simulink model "raven2_model"  (R2015b)
settings: Solver=ode5  SolverMode=SingleTasking  StartTime=0.0  StopTime=19.414  FixedStep=1e-3  RelTol=1e-3
values from neighbouring files (symbols this model uses):
  be1 = 1000*1    (= 1000)    [global_vars.m]
  be2 = 3*1380    (= 4140)    [global_vars.m]
  be3 = 1.0*400    (= 400)    [global_vars.m]
  F_cl1 = 0.505*1    (= 0.505)    [global_vars.m]
  F_cl2 = 0.49*1    (= 0.49)    [global_vars.m]
  F_cl3 = 0.53*10    (= 5.3)    [global_vars.m]
  F_vl1 = 0.00505*1.0    (= 0.00505)    [global_vars.m]
  F_vl2 = 0.0049*1    (= 0.0049)    [global_vars.m]
  F_vl3 = 0.0053*10    (= 0.053)    [global_vars.m]
  I1 = R1*[17.376 0.291 -0.374;0.291 11 -5.483;-0.374 -5.483 6.499]*1e-3*R1'+dI    [global_vars.m]
  I2 = R2*[81.579 0.773 0.762;0.773 44.329 37.973;0.762 37.973 37.686]*1e-3*R2'    [global_vars.m]
  I3 = R3*[2.908 -0.001 -0.066;-0.001 3.009 -0.009;-0.066 -0.009 0.355]*1e-3*R3'    [global_vars.m]
  Im1 = 2.847e-4*1.0    (= 0.0002847)    [global_vars.m]
  Im2 = 2.847e-4    (= 0.0002847)    [global_vars.m]
  Im3 = 2.847e-4    (= 0.0002847)    [global_vars.m]
  j1_r_max = 115/180*pi    (= 2.00712863979)    [joint_limits.m]
  j1_r_min = 10/180*pi    (= 0.174532925199)    [joint_limits.m]
  j2_r_max = 3*pi/4    (= 2.35619449019)    [joint_limits.m]
  j2_r_min = pi/4    (= 0.785398163397)    [joint_limits.m]
  j3_r_max = 520/1000    (= 0.52)    [joint_limits.m]
  j3_r_min = 260/1000    (= 0.26)    [joint_limits.m]
  jl_kd = 0.0    (= 0)    [global_vars.m]
  jl_kp = 0    [global_vars.m]
  kd_arm1 = 0.008*tr_1    (= 1.08957004405)    [global_vars.m]
  kd_arm2 = 20    [global_vars.m]
  kd_arm3 = 200    [global_vars.m]
  ke1 = 720e3    (= 720000)    [global_vars.m]
  ke2 = 3*88e3    (= 264000)    [global_vars.m]
  ke3 = 1*9.25e3    (= 9250)    [global_vars.m]
  ki_arm1 = 0    [global_vars.m]
  ki_arm2 = 0    [global_vars.m]
  ki_arm3 = 0    [global_vars.m]
  kp_arm1 = 0.3*tr_1    (= 40.858876652)    [global_vars.m]
  kp_arm2 = 500    [global_vars.m]
  kp_arm3 = 500    [global_vars.m]
  m1 = 0.503    [global_vars.m]
  m1_pos_ini = mpos1(1)    [initial_config.m]
  m1_vel_ini = mvel1(1)    [initial_config.m]
  m2 = 0.753    [global_vars.m]
  m2_pos_ini = mpos2(1)    [initial_config.m]
  m2_vel_ini = mvel2(1)    [initial_config.m]
  m3 = 0.407    [global_vars.m]
  m3_pos_ini = mpos3(1)    [initial_config.m]
  m3_vel_ini = mvel3(1)    [initial_config.m]
  N = 12.25    [global_vars.m]
  r_l1 = 63.095e-3    (= 0.063095)    [global_vars.m]
  r_l2 = 56.298e-3    (= 0.056298)    [global_vars.m]
  r_l3 = 1    [global_vars.m]
  r_mc1 = 5.675e-3    (= 0.005675)    [global_vars.m]
  r_mc2 = 5.675e-3    (= 0.005675)    [global_vars.m]
  r_mc3 = 5.675e-3    (= 0.005675)    [global_vars.m]
  tau_cm1 = 8.11e-2*0.9    (= 0.07299)    [global_vars.m]
  tau_cm2 = 4.11e-2*1.2    (= 0.04932)    [global_vars.m]
  tau_cm3 = 5.11e-2*2    (= 0.1022)    [global_vars.m]
  tau_vm1 = 1.9e-4*2    (= 0.00038)    [global_vars.m]
  tau_vm2 = 1.8e-4*12    (= 0.00216)    [global_vars.m]
  tau_vm3 = 7.1e-4*2    (= 0.00142)    [global_vars.m]
  theta1_0_r = pi/3    (= 1.0471975512)    [initial_config.m]    (also in main.m = random1*pi/180)
  theta1_d_r = 60*pi/180    (= 1.0471975512)    [main.m]
  theta2_0_r = pi/2    (= 1.57079632679)    [initial_config.m]    (also in main.m = random2*pi/180)
  theta2_d_r = 60*pi/180    (= 1.0471975512)    [main.m]
  theta3_0_r = 500/1000    (= 0.5)    [initial_config.m]    (also in main.m = random3/1000)
  theta3_d_r = 400/1000    (= 0.4)    [main.m]
libraries: mblibv1 x40, simulink x6
settings Model: Creator=raven_lab  LastModifiedBy=raven
settings DataIOCC: SaveFormat=Array
settings OptimizationCC: BlockReduction=off  BooleanDataType=off
settings DebuggingCC: SaveWithParameterizedLinksMsg=none  UnderspecifiedInitializationDetection=Classic  MergeDetectMultiDrivingBlocksExec=none  SignalResolutionControl=TryResolveAllWithWarning  MaskedZcDiagnostic=none  IgnoredZcDiagnostic=none
settings HardwareCC: ProdBitPerPointer=32  ProdLargestAtomicFloat=None  ProdIntDivRoundTo=Undefined  ProdEndianess=Unspecified  ProdWordSize=32  ProdHWDeviceType=32-bit Generic  TargetUnknown=on
settings GRTTargetCC: GeneratePreprocessorConditionals=Disable all
settings ConfigComp: CovModelRefEnable=Off
settings SimMechanicsCC: VisSampleTime=0.033  LastVizWinPosition=[1 41 1920 939]  CamPosition=[-0.0290778;0.260252;12.1482;]  CamTarget=[-0.0290778;0.260252;0.0240561;]  CamUpVector=[0;1;0;]  CamHeight=0.834655  VisBackgroundColor=[0.9;0.9;0.95;]  DefaultBodyColor=[1;0;0;]

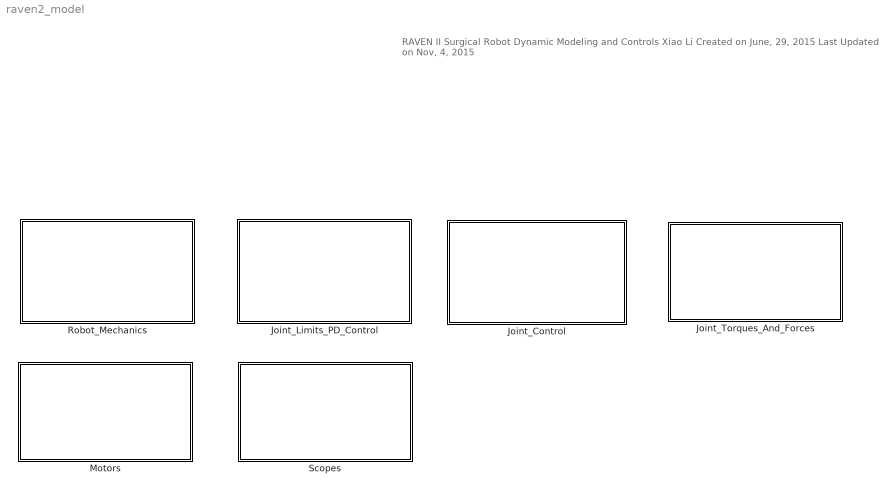
== system raven2_model ==
  note: RAVEN II Surgical Robot
      |
      | Dynamic Modeling and Controls
      |
      | Xiao Li
      |
      | Created on June, 29, 2015
      | Last Updated on Nov, 4, 2015
  Joint_Control : Subsystem
  Joint_Limits_PD_Control : Subsystem
  Joint_Torques_And_Forces : Subsystem
  Motors : Subsystem
  Robot_Mechanics : Subsystem
  Scopes : Subsystem

== system raven2_model/Joint_Control ==
  left_arm_control_command_signal : Subsystem
  right_arm_control_command_signal : Subsystem

== system raven2_model/Joint_Limits_PD_Control ==
  joint_r1_limit : Subsystem
  joint_r2_limit : Subsystem
  joint_r3_limit : Subsystem

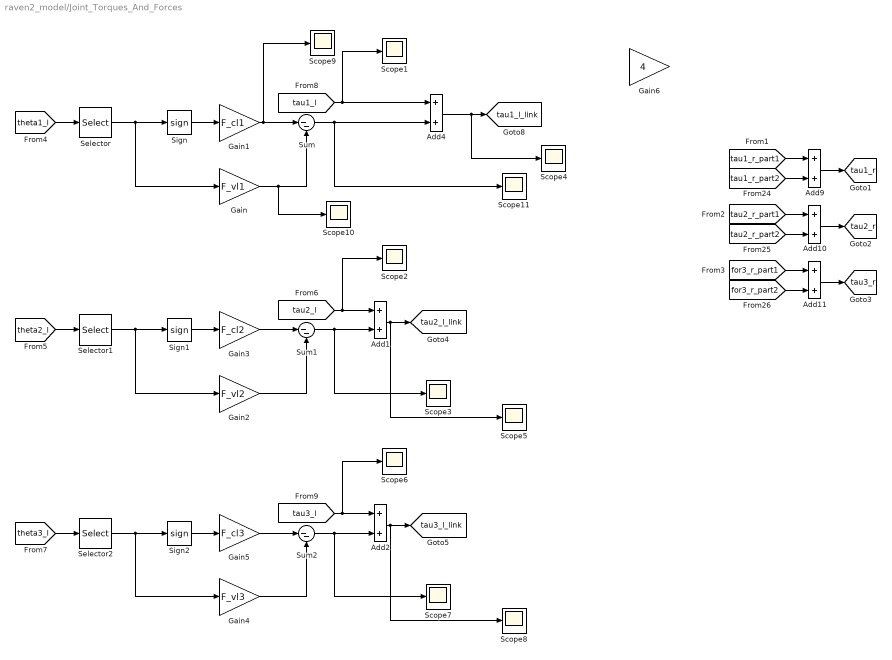
== system raven2_model/Joint_Torques_And_Forces ==
  Add{1..2,4,9..11} (6 alike) : Sum
  Gain : Gain  Gain=F_vl1
  Gain1 : Gain  Gain=F_cl1
  Gain2 : Gain  Gain=F_vl2
  Gain3 : Gain  Gain=F_cl2
  Gain4 : Gain  Gain=F_vl3
  Gain5 : Gain  Gain=F_cl3
  Gain6 : Gain  Gain=4
  Scope{1..11} (11 alike) : Scope
  Selector : Selector  InputPortWidth=2  IndexOptions=Index vector (dialog)  Indices=[2]  OutputSizes=1
  Selector1 : Selector  InputPortWidth=2  IndexOptions=Index vector (dialog)  Indices=[2]  OutputSizes=1
  Selector2 : Selector  InputPortWidth=2  IndexOptions=Index vector (dialog)  Indices=[2]  OutputSizes=1
  Sign : Signum
  Sign1 : Signum
  Sign2 : Signum
  Sum : Sum  Inputs=|--
  Sum1 : Sum  Inputs=|--
  Sum2 : Sum  Inputs=|--
  tag scope: tau1_l_link=global, tau1_r=global, tau2_l_link=global, tau2_r=global, tau3_l_link=global, tau3_r=global
  wires:
  Add4/1 -> Scope4/1, [tau1_l_link]
  [tau1_r_part2] -> Add9/2
  Add9/1 -> [tau1_r]
  [tau2_r_part2] -> Add10/2
  Add10/1 -> [tau2_r]
  [for3_r_part2] -> Add11/2
  Add11/1 -> [tau3_r]
  [tau1_r_part1] -> Add9/1
  [tau2_r_part1] -> Add10/1
  [for3_r_part1] -> Add11/1
  [theta1_l] -> Selector/1
  Sign/1 -> Gain1/1
  Selector/1 -> Gain/1, Sign/1
  Gain1/1 -> Scope9/1, Sum/1
  Gain/1 -> Scope10/1, Sum/2
  Sum/1 -> Scope11/1, Add4/2
  Add1/1 -> Scope5/1, [tau2_l_link]
  [theta2_l] -> Selector1/1
  Sign1/1 -> Gain3/1
  Selector1/1 -> Gain2/1, Sign1/1
  Gain3/1 -> Sum1/1
  Gain2/1 -> Sum1/2
  Sum1/1 -> Scope3/1, Add1/2
  [tau2_l] -> Scope2/1, Add1/1
  Add2/1 -> Scope8/1, [tau3_l_link]
  [theta3_l] -> Selector2/1
  Sign2/1 -> Gain5/1
  Selector2/1 -> Gain4/1, Sign2/1
  Gain5/1 -> Sum2/1
  Gain4/1 -> Sum2/2
  Sum2/1 -> Scope7/1, Add2/2
  [tau3_l] -> Scope6/1, Add2/1
  [tau1_l] -> Add4/1, Scope1/1

== system raven2_model/Motors ==
  Motor1 : Subsystem
  Motor2 : Subsystem
  Motor3 : Subsystem

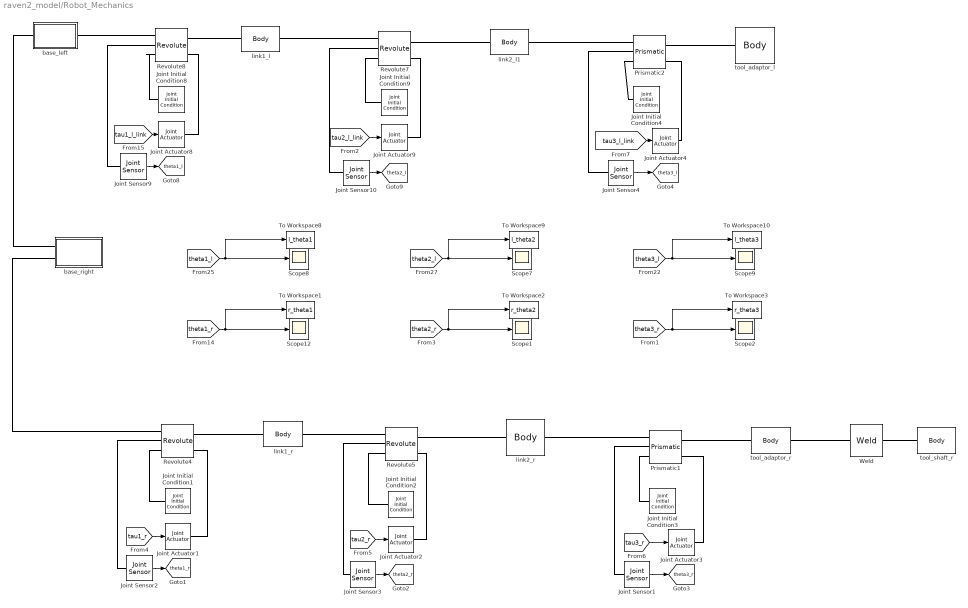
== system raven2_model/Robot_Mechanics ==
  Joint Actuator{1..2,8..9} (4 alike) : mblibv1/Sensors &  Actuators/Joint Actuator  UpdateFromCAD=off  PhysicalDomain=Mechanical  PortType=blob  ActuationStyle=Force  AngleUnits=deg  ArcVelocityUnits=deg/s  ArcAccelerationUnits=deg/s^2  CoordPositionUnits=m  VelocityUnits=m/s  AccelerationUnits=m/s^2  ForceUnits=N  TorqueUnits=N*m  ActiveIO=on  Width=1  DialogClass=MechanicalActuatorBlock  Primitive=R1  ReferenceFrame=Absolute (World)
  Joint Actuator3 : mblibv1/Sensors &  Actuators/Joint Actuator  UpdateFromCAD=off  PhysicalDomain=Mechanical  PortType=blob  ActuationStyle=Force  AngleUnits=deg  ArcVelocityUnits=deg/s  ArcAccelerationUnits=deg/s^2  CoordPositionUnits=m  VelocityUnits=m/s  AccelerationUnits=m/s^2  ForceUnits=N  TorqueUnits=N*m  ActiveIO=on  Width=1  DialogClass=MechanicalActuatorBlock  Primitive=P1  ReferenceFrame=Absolute (World)
  Joint Actuator4 : mblibv1/Sensors &  Actuators/Joint Actuator  UpdateFromCAD=off  PhysicalDomain=Mechanical  PortType=blob  ActuationStyle=Force  AngleUnits=deg  ArcVelocityUnits=deg/s  ArcAccelerationUnits=deg/s^2  CoordPositionUnits=m  VelocityUnits=m/s  AccelerationUnits=m/s^2  ForceUnits=N  TorqueUnits=N*m  ActiveIO=on  Width=1  DialogClass=MechanicalActuatorBlock  Primitive=P1  ReferenceFrame=Absolute (World)
  Joint Initial Condition1 : mblibv1/Sensors &  Actuators/Joint Initial Condition  UpdateFromCAD=off  LeftPortType=blob  RightPortType=blob  PhysicalDomain=mechanical  DialogClass=InitialConditionBlock  InitialConditions=P1$false$0$m$deg$0$m/s$deg/s#P2$false$0$m$deg$0$m/s$deg/s#P3$false$0$m$deg$0$m/s$deg/s#R1$true$theta1_0_r$m$rad$theta1_d_0_r$m/s$rad/s#R2$false$0$m$deg$0$m/s$deg/s#R3$false$0$m$deg$0$m/s$deg/s#S$false$0$m$deg$0$m/s$deg/s  P1PIC=0  P1VIC=0  P2PIC=0  P2VIC=0  P3PIC=0  P3VIC=0  R1PIC=theta1_0_r  R1VIC=theta1_d_0_r  R2PIC=0  R2VIC=0  R3PIC=0  R3VIC=0  SPIC=0  SVIC=0
  Joint Initial Condition2 : mblibv1/Sensors &  Actuators/Joint Initial Condition  UpdateFromCAD=off  LeftPortType=blob  RightPortType=blob  PhysicalDomain=mechanical  DialogClass=InitialConditionBlock  InitialConditions=P1$false$0$m$deg$0$m/s$deg/s#P2$false$0$m$deg$0$m/s$deg/s#P3$false$0$m$deg$0$m/s$deg/s#R1$true$theta2_0_r$m$rad$theta2_d_0_r$m/s$rad/s#R2$false$0$m$deg$0$m/s$deg/s#R3$false$0$m$deg$0$m/s$deg/s#S$false$0$m$deg$0$m/s$deg/s  P1PIC=0  P1VIC=0  P2PIC=0  P2VIC=0  P3PIC=0  P3VIC=0  R1PIC=theta2_0_r  R1VIC=theta2_d_0_r  R2PIC=0  R2VIC=0  R3PIC=0  R3VIC=0  SPIC=0  SVIC=0
  Joint Initial Condition3 : mblibv1/Sensors &  Actuators/Joint Initial Condition  UpdateFromCAD=off  LeftPortType=blob  RightPortType=blob  PhysicalDomain=mechanical  DialogClass=InitialConditionBlock  InitialConditions=P1$true$theta3_0_r$m$deg$theta3_d_0_r$m/s$deg/s#P2$false$0$m$deg$0$m/s$deg/s#P3$false$0$m$deg$0$m/s$deg/s#R1$false$theta2_0_r$m$rad$0$m/s$rad/s#R2$false$0$m$deg$0$m/s$deg/s#R3$false$0$m$deg$0$m/s$deg/s#S$false$0$m$deg$0$m/s$deg/s  P1PIC=theta3_0_r  P1VIC=theta3_d_0_r  P2PIC=0  P2VIC=0  P3PIC=0  P3VIC=0  R1PIC=0  R1VIC=0  R2PIC=0  R2VIC=0  R3PIC=0  R3VIC=0  SPIC=0  SVIC=0
  Joint Initial Condition4 : mblibv1/Sensors &  Actuators/Joint Initial Condition  UpdateFromCAD=off  LeftPortType=blob  RightPortType=blob  PhysicalDomain=mechanical  DialogClass=InitialConditionBlock  InitialConditions=P1$true$theta3_0_l$m$deg$theta3_d_0_l$m/s$deg/s#P2$false$0$m$deg$0$m/s$deg/s#P3$false$0$m$deg$0$m/s$deg/s#R1$false$theta2_0_r$m$rad$0$m/s$rad/s#R2$false$0$m$deg$0$m/s$deg/s#R3$false$0$m$deg$0$m/s$deg/s#S$false$0$m$deg$0$m/s$deg/s  P1PIC=theta3_0_l  P1VIC=theta3_d_0_l  P2PIC=0  P2VIC=0  P3PIC=0  P3VIC=0  R1PIC=0  R1VIC=0  R2PIC=0  R2VIC=0  R3PIC=0  R3VIC=0  SPIC=0  SVIC=0
  Joint Initial Condition8 : mblibv1/Sensors &  Actuators/Joint Initial Condition  UpdateFromCAD=off  LeftPortType=blob  RightPortType=blob  PhysicalDomain=mechanical  DialogClass=InitialConditionBlock  InitialConditions=P1$false$0$m$deg$0$m/s$deg/s#P2$false$0$m$deg$0$m/s$deg/s#P3$false$0$m$deg$0$m/s$deg/s#R1$true$theta1_0_l$m$rad$theta1_d_0_l$m/s$rad/s#R2$false$0$m$deg$0$m/s$deg/s#R3$false$0$m$deg$0$m/s$deg/s#S$false$0$m$deg$0$m/s$deg/s  P1PIC=0  P1VIC=0  P2PIC=0  P2VIC=0  P3PIC=0  P3VIC=0  R1PIC=theta1_0_l  R1VIC=theta1_d_0_l  R2PIC=0  R2VIC=0  R3PIC=0  R3VIC=0  SPIC=0  SVIC=0
  Joint Initial Condition9 : mblibv1/Sensors &  Actuators/Joint Initial Condition  UpdateFromCAD=off  LeftPortType=blob  RightPortType=blob  PhysicalDomain=mechanical  DialogClass=InitialConditionBlock  InitialConditions=P1$false$0$m$deg$0$m/s$deg/s#P2$false$0$m$deg$0$m/s$deg/s#P3$false$0$m$deg$0$m/s$deg/s#R1$true$theta2_0_l$m$rad$theta2_d_0_l$m/s$rad/s#R2$false$0$m$deg$0$m/s$deg/s#R3$false$0$m$deg$0$m/s$deg/s#S$false$0$m$deg$0$m/s$deg/s  P1PIC=0  P1VIC=0  P2PIC=0  P2VIC=0  P3PIC=0  P3VIC=0  R1PIC=theta2_0_l  R1VIC=theta2_d_0_l  R2PIC=0  R2VIC=0  R3PIC=0  R3VIC=0  SPIC=0  SVIC=0
  Joint Sensor1 : mblibv1/Sensors &  Actuators/Joint Sensor  UpdateFromCAD=off  PhysicalDomain=Mechanical  PortType=blob  Muxed=on  Pose=off  Angle=on  AngleUnits=deg  ArcVelocity=on  ArcVelocityUnits=deg/s  ArcAcceleration=off  ArcAccelerationUnits=deg/s^2  CoordPosition=on  CoordPositionUnits=m  Velocity=on  VelocityUnits=m/s  Acceleration=off  AccelerationUnits=m/s^2  Quaternion=on  QuaternionDT=off  QuaternionDDT=off  QuaternionUnits=off  OutputVector=[1]  ActiveIO=on  Width=2  DialogClass=MechanicalSensorBlock  Primitive=P1  Force=off  ForceUnits=N  Torque=off  TorqueUnits=N*m  ReferenceFrame=Absolute (World)  ReactionSensedSide=Base  ReactionReferenceFrame=Absolute (World)  ReactionForce=off  ReactionForceUnits=N  ReactionMoment=off  ReactionMomentUnits=N*m
  Joint Sensor{2..3,9..10} (4 alike) : mblibv1/Sensors &  Actuators/Joint Sensor  UpdateFromCAD=off  PhysicalDomain=Mechanical  PortType=blob  Muxed=on  Pose=off  Angle=on  AngleUnits=rad  ArcVelocity=on  ArcVelocityUnits=rad/s  ArcAcceleration=off  ArcAccelerationUnits=deg/s^2  CoordPosition=on  CoordPositionUnits=m  Velocity=off  VelocityUnits=m/s  Acceleration=off  AccelerationUnits=m/s^2  Quaternion=on  QuaternionDT=off  QuaternionDDT=off  QuaternionUnits=off  OutputVector=[1]  ActiveIO=on  Width=2  DialogClass=MechanicalSensorBlock  Primitive=R1  Force=off  ForceUnits=N  Torque=off  TorqueUnits=N*m  ReferenceFrame=Absolute (World)  ReactionSensedSide=Base  ReactionReferenceFrame=Absolute (World)  ReactionForce=off  ReactionForceUnits=N  ReactionMoment=off  ReactionMomentUnits=N*m
  Joint Sensor4 : mblibv1/Sensors &  Actuators/Joint Sensor  UpdateFromCAD=off  PhysicalDomain=Mechanical  PortType=blob  Muxed=on  Pose=off  Angle=on  AngleUnits=deg  ArcVelocity=on  ArcVelocityUnits=deg/s  ArcAcceleration=off  ArcAccelerationUnits=deg/s^2  CoordPosition=on  CoordPositionUnits=m  Velocity=on  VelocityUnits=m/s  Acceleration=off  AccelerationUnits=m/s^2  Quaternion=on  QuaternionDT=off  QuaternionDDT=off  QuaternionUnits=off  OutputVector=[1]  ActiveIO=on  Width=2  DialogClass=MechanicalSensorBlock  Primitive=P1  Force=off  ForceUnits=N  Torque=off  TorqueUnits=N*m  ReferenceFrame=Absolute (World)  ReactionSensedSide=Base  ReactionReferenceFrame=Absolute (World)  ReactionForce=off  ReactionForceUnits=N  ReactionMoment=off  ReactionMomentUnits=N*m
  Prismatic1 : mblibv1/Joints/Prismatic  LConnTagsString=__newl0|SA1|SA2  RConnTagsString=__newr0|SA1  UpdateFromCAD=on  NumSAPorts=3  CutJoint=off  MarkAsCut=off  Primitives=prismatic  PrimitiveProps=P1$World$-[0.601815,0,0.798636]$prismatic  DialogClass=JointBlock  P1Axis=-[0.601815,0,0.798636]
  Prismatic2 : mblibv1/Joints/Prismatic  LConnTagsString=__newl0|SA1|SA2  RConnTagsString=__newr0|SA1  UpdateFromCAD=on  NumSAPorts=3  CutJoint=off  MarkAsCut=off  Primitives=prismatic  PrimitiveProps=P1$World$-[0.920505,0,-0.390731]$prismatic  DialogClass=JointBlock  P1Axis=-[0.920505,0,-0.390731]
  Revolute4 : mblibv1/Joints/Revolute  LConnTagsString=__newl0|SA1|SA2  RConnTagsString=__newr0|SA1  UpdateFromCAD=on  NumSAPorts=3  CutJoint=off  MarkAsCut=off  Primitives=prismatic  PrimitiveProps=R1$World$[1,0,0]$revolute  DialogClass=JointBlock  R1Axis=[1,0,0]
  Revolute5 : mblibv1/Joints/Revolute  LConnTagsString=__newl0|SA1|SA2  RConnTagsString=__newr0|SA1  UpdateFromCAD=on  NumSAPorts=3  CutJoint=off  MarkAsCut=off  Primitives=prismatic  PrimitiveProps=R1$World$-[-0.258819,0,0.965926]$revolute  DialogClass=JointBlock  R1Axis=-[-0.258819,0,0.965926]
  Revolute7 : mblibv1/Joints/Revolute  LConnTagsString=__newl0|SA1|SA2  RConnTagsString=__newr0|SA1  UpdateFromCAD=on  NumSAPorts=3  CutJoint=off  MarkAsCut=off  Primitives=prismatic  PrimitiveProps=R1$World$-[-0.258819,0,0.965926]$revolute  DialogClass=JointBlock  R1Axis=-[-0.258819,0,0.965926]
  Revolute8 : mblibv1/Joints/Revolute  LConnTagsString=__newl0|SA1|SA2  RConnTagsString=__newr0|SA1  UpdateFromCAD=on  NumSAPorts=3  CutJoint=off  MarkAsCut=off  Primitives=prismatic  PrimitiveProps=R1$World$[1,0,0]$revolute  DialogClass=JointBlock  R1Axis=[1,0,0]
  Scope{1..2,7..9,12} (6 alike) : Scope
  To Workspace1 : ToWorkspace  VariableName=r_theta1  SaveFormat=Timeseries  SampleTime=-1
  To Workspace10 : ToWorkspace  VariableName=l_theta3  SaveFormat=Timeseries  SampleTime=-1
  To Workspace2 : ToWorkspace  VariableName=r_theta2  SaveFormat=Timeseries  SampleTime=-1
  To Workspace3 : ToWorkspace  VariableName=r_theta3  SaveFormat=Timeseries  SampleTime=-1
  To Workspace8 : ToWorkspace  VariableName=l_theta1  SaveFormat=Timeseries  SampleTime=-1
  To Workspace9 : ToWorkspace  VariableName=l_theta2  SaveFormat=Timeseries  SampleTime=-1
  Weld : mblibv1/Joints/Weld  LConnTagsString=__newl0  RConnTagsString=__newr0  UpdateFromCAD=off  NumSAPorts=0  CutJoint=off  MarkAsCut=off  Primitives=weld  PrimitiveProps=W$WORLD$[0 0 0]$weld  DialogClass=JointBlock  WAxis=[0 0 0]
  base_left : Subsystem
  base_right : Subsystem
  link1_l : mblibv1/Bodies/Body  LConnTagsString=CS3  RConnTagsString=CS2  UpdateFromCAD=on  DialogClass=MechanicalBodyBlock  Mass=m1  MassUnits=kg  InertiaUnits=kg*m^2  Inertia=I1  Shape=Cylinder  ShapeDims=[1 1]  ShapeUnits=m  ShapeUse=false  Density=1  DensityUnits=kg/m^3  DensityUse=false  GraphicsMode=GFXFILE  GraphicsFileName=full_robot - Sim_R2-Link1-L-1.STL  BodyColorSelMode=COLORPALETTE  BodyColor=[0.49412 0.49412 0.49412]  AttachedToCS=CS1  CG=Right$CG$[-0.215224 0.00717636 0.104721]$WORLD$WORLD$m$[1 0 0;0 -1 0;0 0 -1]$3x3 Transform$rad$WORLD$false$none  WorkingFrames=Right$CS1$[-0.278513 0 0]$WORLD$WORLD$m$[1 0 0;0 -1 0;0 0 -1]$3x3 Transform$rad$WORLD$false$none#Right$CS2$[-0.121275 0 0.143591]$WORLD$WORLD$m$[1 0 0;0 1 0;0 0 1]$3x3 Transform$rad$WORLD$true$none#Left$CS3$[-0.284078 0 0]$WORLD$WORLD$m$[1 0 0;0 1 0;0 0 1]$3x3 Transform$rad$WORLD$true$none  CGPos=[-0.215224 0.00717636 0.104721]  CGRot=[1 0 0;0 -1 0;0 0 -1]  CS0Pos=[]  CS0Rot=[]  CS1Pos=[-0.278513 0 0]  CS1Rot=[1 0 0;0 -1 0;0 0 -1]  CS2Pos=[-0.121275 0 0.143591]  CS2Rot=[1 0 0;0 1 0;0 0 1]  CS3Pos=[-0.284078 0 0]  CS3Rot=[1 0 0;0 1 0;0 0 1]  CS4Pos=[]  CS4Rot=[]  CS5Pos=[]  CS5Rot=[]  CS6Pos=[]  CS6Rot=[]  CS7Pos=[]  CS7Rot=[]  CS8Pos=[]  CS8Rot=[]  CS9Pos=[]  CS9Rot=[]  CS10Pos=[]  CS10Rot=[]  CS11Pos=[]  CS11Rot=[]  CS12Pos=[]  CS12Rot=[]  CS13Pos=[]  CS13Rot=[]  CS14Pos=[]  CS14Rot=[]  CS15Pos=[]  CS15Rot=[]  CS16Pos=[]  CS16Rot=[]  CS17Pos=[]  CS17Rot=[]  CS18Pos=[]  CS18Rot=[]  CS19Pos=[]  CS19Rot=[]  CS20Pos=[]  CS20Rot=[]
  link1_r : mblibv1/Bodies/Body  LConnTagsString=CS2  RConnTagsString=CS3  UpdateFromCAD=on  DialogClass=MechanicalBodyBlock  Mass=0.307878  MassUnits=kg  InertiaUnits=kg*m^2  Inertia=[0.000865925,5.99521e-06,-0.000512747;5.99521e-06,0.00142355,-6.10689e-06;-0.000512747,-6.10689e-06,0.000580565]  Shape=Cylinder  ShapeDims=[1 1]  ShapeUnits=m  ShapeUse=false  Density=1  DensityUnits=kg/m^3  DensityUse=false  GraphicsMode=GFXFILE  GraphicsFileName=full_robot - Sim_R2-Link1-R-1.STL  BodyColorSelMode=COLORPALETTE  BodyColor=[0.494118;0.494118;0.494118]  AttachedToCS=CS1  CG=Right$CG$[0.132424 -0.00717684 -0.104721]$WORLD$WORLD$m$[1 0 0;0 1 0;0 0 1]$3x3 Transform$rad$WORLD$false$none  WorkingFrames=Right$CS1$[0.195713 0 0]$WORLD$WORLD$m$[1 0 0;0 1 0;0 0 1]$3x3 Transform$rad$WORLD$false$none#Left$CS2$[0.200746 0 0]$WORLD$WORLD$m$[1 0 0;0 1 0;0 0 1]$3x3 Transform$rad$WORLD$true$none#Right$CS3$[0.0384751 0 -0.143591]$WORLD$WORLD$m$[1 0 0;0 1 0;0 0 1]$3x3 Transform$rad$WORLD$true$none  CGPos=[0.132424 -0.00717684 -0.104721]  CGRot=[1 0 0;0 1 0;0 0 1]  CS0Pos=[]  CS0Rot=[]  CS1Pos=[0.195713 0 0]  CS1Rot=[1 0 0;0 1 0;0 0 1]  CS2Pos=[0.200746 0 0]  CS2Rot=[1 0 0;0 1 0;0 0 1]  CS3Pos=[0.0384751 0 -0.143591]  CS3Rot=[1 0 0;0 1 0;0 0 1]  CS4Pos=[]  CS4Rot=[]  CS5Pos=[]  CS5Rot=[]  CS6Pos=[]  CS6Rot=[]  CS7Pos=[]  CS7Rot=[]  CS8Pos=[]  CS8Rot=[]  CS9Pos=[]  CS9Rot=[]  CS10Pos=[]  CS10Rot=[]  CS11Pos=[]  CS11Rot=[]  CS12Pos=[]  CS12Rot=[]  CS13Pos=[]  CS13Rot=[]  CS14Pos=[]  CS14Rot=[]  CS15Pos=[]  CS15Rot=[]  CS16Pos=[]  CS16Rot=[]  CS17Pos=[]  CS17Rot=[]  CS18Pos=[]  CS18Rot=[]  CS19Pos=[]  CS19Rot=[]  CS20Pos=[]  CS20Rot=[]
  link2_l1 : mblibv1/Bodies/Body  LConnTagsString=CS3  RConnTagsString=CS2  UpdateFromCAD=on  DialogClass=MechanicalBodyBlock  Mass=m2  MassUnits=kg  InertiaUnits=kg*m^2  Inertia=I2  Shape=Cylinder  ShapeDims=[1 1]  ShapeUnits=m  ShapeUse=false  Density=1  DensityUnits=kg/m^3  DensityUse=false  GraphicsMode=GFXFILE  GraphicsFileName=full_robot - Sim_R2-Link2-L-1.STL  BodyColorSelMode=COLORPALETTE  BodyColor=[0 0.44706 0.74118]  AttachedToCS=CS1  CG=Right$CG$[-0.30597 -0.00410333 0.168286]$WORLD$WORLD$m$[0.258819 -0.965926 0;0 0 1;-0.965926 -0.258819 0]$3x3 Transform$rad$WORLD$false$none  WorkingFrames=Right$CS1$[-0.162302 -0.0075 0.179517]$WORLD$WORLD$m$[0.258819 -0.965926 0;0 0 1;-0.965926 -0.258819 0]$3x3 Transform$rad$WORLD$false$none#Right$CS2$[-0.209463 0 0.0537709]$WORLD$WORLD$m$[1 0 0;0 1 0;0 0 1]$3x3 Transform$rad$WORLD$true$none#Left$CS3$[-0.121275 0 0.143591]$WORLD$WORLD$m$[1 0 0;0 1 0;0 0 1]$3x3 Transform$rad$WORLD$true$none  CGPos=[-0.30597 -0.00410333 0.168286]  CGRot=[0.258819 -0.965926 0;0 0 1;-0.965926 -0.258819 0]  CS0Pos=[]  CS0Rot=[]  CS1Pos=[-0.162302 -0.0075 0.179517]  CS1Rot=[0.258819 -0.965926 0;0 0 1;-0.965926 -0.258819 0]  CS2Pos=[-0.209463 0 0.0537709]  CS2Rot=[1 0 0;0 1 0;0 0 1]  CS3Pos=[-0.121275 0 0.143591]  CS3Rot=[1 0 0;0 1 0;0 0 1]  CS4Pos=[]  CS4Rot=[]  CS5Pos=[]  CS5Rot=[]  CS6Pos=[]  CS6Rot=[]  CS7Pos=[]  CS7Rot=[]  CS8Pos=[]  CS8Rot=[]  CS9Pos=[]  CS9Rot=[]  CS10Pos=[]  CS10Rot=[]  CS11Pos=[]  CS11Rot=[]  CS12Pos=[]  CS12Rot=[]  CS13Pos=[]  CS13Rot=[]  CS14Pos=[]  CS14Rot=[]  CS15Pos=[]  CS15Rot=[]  CS16Pos=[]  CS16Rot=[]  CS17Pos=[]  CS17Rot=[]  CS18Pos=[]  CS18Rot=[]  CS19Pos=[]  CS19Rot=[]  CS20Pos=[]  CS20Rot=[]
  link2_r : mblibv1/Bodies/Body  LConnTagsString=CS2  RConnTagsString=CS3  UpdateFromCAD=on  DialogClass=MechanicalBodyBlock  Mass=0.298287  MassUnits=kg  InertiaUnits=kg*m^2  Inertia=[0.00536881,-0.00335802,0.000118788;-0.00335802,0.00241011,0.000122449;0.000118788,0.000122449,0.00763968]  Shape=Cylinder  ShapeDims=[1 1]  ShapeUnits=m  ShapeUse=false  Density=1  DensityUnits=kg/m^3  DensityUse=false  GraphicsMode=GFXFILE  GraphicsFileName=full_robot - Sim_R2-Link2-R-1.STL  BodyColorSelMode=COLORPALETTE  BodyColor=[0;0.447059;0.741176]  AttachedToCS=CS1  CG=Right$CG$[-0.109127 -0.00410285 -0.257322]$WORLD$WORLD$m$[0.258819 -0.965926 0;0 0 1;-0.965926 -0.258819 0]$3x3 Transform$rad$WORLD$false$none  WorkingFrames=Right$CS1$[0.020908 -0.0075 -0.195217]$WORLD$WORLD$m$[0.258819 -0.965926 0;0 0 1;-0.965926 -0.258819 0]$3x3 Transform$rad$WORLD$false$none#Left$CS2$[0.0384751 0 -0.143591]$WORLD$WORLD$m$[1 0 0;0 1 0;0 0 1]$3x3 Transform$rad$WORLD$true$none#Right$CS3$[-0.0828081 0 -0.109899]$WORLD$WORLD$m$[1 0 0;0 1 0;0 0 1]$3x3 Transform$rad$WORLD$true$none  CGPos=[-0.109127 -0.00410285 -0.257322]  CGRot=[0.258819 -0.965926 0;0 0 1;-0.965926 -0.258819 0]  CS0Pos=[]  CS0Rot=[]  CS1Pos=[0.020908 -0.0075 -0.195217]  CS1Rot=[0.258819 -0.965926 0;0 0 1;-0.965926 -0.258819 0]  CS2Pos=[0.0384751 0 -0.143591]  CS2Rot=[1 0 0;0 1 0;0 0 1]  CS3Pos=[-0.0828081 0 -0.109899]  CS3Rot=[1 0 0;0 1 0;0 0 1]  CS4Pos=[]  CS4Rot=[]  CS5Pos=[]  CS5Rot=[]  CS6Pos=[]  CS6Rot=[]  CS7Pos=[]  CS7Rot=[]  CS8Pos=[]  CS8Rot=[]  CS9Pos=[]  CS9Rot=[]  CS10Pos=[]  CS10Rot=[]  CS11Pos=[]  CS11Rot=[]  CS12Pos=[]  CS12Rot=[]  CS13Pos=[]  CS13Rot=[]  CS14Pos=[]  CS14Rot=[]  CS15Pos=[]  CS15Rot=[]  CS16Pos=[]  CS16Rot=[]  CS17Pos=[]  CS17Rot=[]  CS18Pos=[]  CS18Rot=[]  CS19Pos=[]  CS19Rot=[]  CS20Pos=[]  CS20Rot=[]
  tool_adaptor_l : mblibv1/Bodies/Body  RConnTagsString=CS3  UpdateFromCAD=on  DialogClass=MechanicalBodyBlock  Mass=m3  MassUnits=kg  InertiaUnits=kg*m^2  Inertia=I3  Shape=Cylinder  ShapeDims=[1 1]  ShapeUnits=m  ShapeUse=false  Density=1  DensityUnits=kg/m^3  DensityUse=false  GraphicsMode=GFXFILE  GraphicsFileName=full_robot - tool_adaptor_r-3.STL  BodyColorSelMode=COLORPALETTE  BodyColor=[1 1 0]  AttachedToCS=CS1  CG=Right$CG$[-0.0750172 0.000150527 0.0170169]$WORLD$WORLD$m$[0 -0.920505 -0.390731;-1 0 0;0 0.390731 -0.920505]$3x3 Transform$rad$WORLD$false$none  WorkingFrames=Right$CS1$[0.0371929 0.0207212 0.0861524]$WORLD$WORLD$m$[0 -0.920505 -0.390731;-1 0 0;0 0.390731 -0.920505]$3x3 Transform$rad$WORLD$false$none#Left$CS2$[-0.0247371 0 -0.0246407]$WORLD$WORLD$m$[1 0 0;0 1 0;0 0 1]$3x3 Transform$rad$WORLD$false$none#Right$CS3$[-0.0303586 0 -0.0222545]$WORLD$WORLD$m$[1 0 0;0 1 0;0 0 1]$3x3 Transform$rad$WORLD$true$none  CGPos=[-0.0750172 0.000150527 0.0170169]  CGRot=[0 -0.920505 -0.390731;-1 0 0;0 0.390731 -0.920505]  CS0Pos=[]  CS0Rot=[]  CS1Pos=[0.0371929 0.0207212 0.0861524]  CS1Rot=[0 -0.920505 -0.390731;-1 0 0;0 0.390731 -0.920505]  CS2Pos=[-0.0247371 0 -0.0246407]  CS2Rot=[1 0 0;0 1 0;0 0 1]  CS3Pos=[-0.0303586 0 -0.0222545]  CS3Rot=[1 0 0;0 1 0;0 0 1]  CS4Pos=[]  CS4Rot=[]  CS5Pos=[]  CS5Rot=[]  CS6Pos=[]  CS6Rot=[]  CS7Pos=[]  CS7Rot=[]  CS8Pos=[]  CS8Rot=[]  CS9Pos=[]  CS9Rot=[]  CS10Pos=[]  CS10Rot=[]  CS11Pos=[]  CS11Rot=[]  CS12Pos=[]  CS12Rot=[]  CS13Pos=[]  CS13Rot=[]  CS14Pos=[]  CS14Rot=[]  CS15Pos=[]  CS15Rot=[]  CS16Pos=[]  CS16Rot=[]  CS17Pos=[]  CS17Rot=[]  CS18Pos=[]  CS18Rot=[]  CS19Pos=[]  CS19Rot=[]  CS20Pos=[]  CS20Rot=[]
  tool_adaptor_r : mblibv1/Bodies/Body  LConnTagsString=CS3  RConnTagsString=CS2  UpdateFromCAD=on  DialogClass=MechanicalBodyBlock  Mass=0.17959  MassUnits=kg  InertiaUnits=kg*m^2  Inertia=1e3*[1.75049e-07,2.47824e-09,4.64456e-10;2.47824e-09,7.90471e-08,4.11989e-09;4.64456e-10,4.11989e-09,1.78166e-07]  Shape=Cylinder  ShapeDims=[1 1]  ShapeUnits=m  ShapeUse=false  Density=1  DensityUnits=kg/m^3  DensityUse=false  GraphicsMode=GFXFILE  GraphicsFileName=full_robot - tool_adaptor_r-2.STL  BodyColorSelMode=COLORPALETTE  BodyColor=[0;1;0]  AttachedToCS=CS1  CG=Right$CG$[0.0152555 -0.000150527 -0.0108364]$WORLD$WORLD$m$[0 -0.601815 -0.798636;1 0 0;0 -0.798636 0.601815]$3x3 Transform$rad$WORLD$false$none  WorkingFrames=Right$CS1$[0.147 -0.0207212 -0.0146044]$WORLD$WORLD$m$[0 -0.601815 -0.798636;1 0 0;0 -0.798636 0.601815]$3x3 Transform$rad$WORLD$false$none#Right$CS2$[0.0379706 0 0.0503802]$WORLD$WORLD$m$[1 0 0;0 1 0;0 0 1]$3x3 Transform$rad$WORLD$true$none#Left$CS3$[0.0342953 0 0.0455029]$WORLD$WORLD$m$[1 0 0;0 1 0;0 0 1]$3x3 Transform$rad$WORLD$true$none  CGPos=[0.0152555 -0.000150527 -0.0108364]  CGRot=[0 -0.601815 -0.798636;1 0 0;0 -0.798636 0.601815]  CS0Pos=[]  CS0Rot=[]  CS1Pos=[0.147 -0.0207212 -0.0146044]  CS1Rot=[0 -0.601815 -0.798636;1 0 0;0 -0.798636 0.601815]  CS2Pos=[0.0379706 0 0.0503802]  CS2Rot=[1 0 0;0 1 0;0 0 1]  CS3Pos=[0.0342953 0 0.0455029]  CS3Rot=[1 0 0;0 1 0;0 0 1]  CS4Pos=[]  CS4Rot=[]  CS5Pos=[]  CS5Rot=[]  CS6Pos=[]  CS6Rot=[]  CS7Pos=[]  CS7Rot=[]  CS8Pos=[]  CS8Rot=[]  CS9Pos=[]  CS9Rot=[]  CS10Pos=[]  CS10Rot=[]  CS11Pos=[]  CS11Rot=[]  CS12Pos=[]  CS12Rot=[]  CS13Pos=[]  CS13Rot=[]  CS14Pos=[]  CS14Rot=[]  CS15Pos=[]  CS15Rot=[]  CS16Pos=[]  CS16Rot=[]  CS17Pos=[]  CS17Rot=[]  CS18Pos=[]  CS18Rot=[]  CS19Pos=[]  CS19Rot=[]  CS20Pos=[]  CS20Rot=[]
  tool_shaft_r : mblibv1/Bodies/Body  LConnTagsString=CS3  UpdateFromCAD=on  DialogClass=MechanicalBodyBlock  Mass=0.031894  MassUnits=kg  InertiaUnits=kg*m^2  Inertia=[0.000438543,1.00962e-12,-5.16101e-11;1.00962e-12,0.000438544,-2.93392e-12;-5.16101e-11,-2.93392e-12,3.98541e-07]  Shape=Cylinder  ShapeDims=[1 1]  ShapeUnits=m  ShapeUse=false  Density=1  DensityUnits=kg/m^3  DensityUse=false  GraphicsMode=GFXFILE  GraphicsFileName=full_robot - Sim_ToolShaft-1.STL  BodyColorSelMode=COLORPALETTE  BodyColor=[0.79216 0.81961 0.93333]  AttachedToCS=CS1  CG=Right$CG$[0.160168 -1.00252e-08 0.212541]$WORLD$WORLD$m$[0 0.798636 -0.601815;1 0 0;0 -0.601815 -0.798636]$3x3 Transform$rad$WORLD$false$none  WorkingFrames=Right$CS1$[0.278697 0 0.369834]$WORLD$WORLD$m$[0 0.798636 -0.601815;1 0 0;0 -0.601815 -0.798636]$3x3 Transform$rad$WORLD$false$none#Right$CS2$[0.28303 0.0011 0.375585]$WORLD$WORLD$m$[1 0 0;0 1 0;0 0 1]$3x3 Transform$rad$WORLD$false$none#Left$CS3$[0.0379706 0 0.0503802]$WORLD$WORLD$m$[1 0 0;0 1 0;0 0 1]$3x3 Transform$rad$WORLD$true$none  CGPos=[0.160168 -1.00252e-08 0.212541]  CGRot=[0 0.798636 -0.601815;1 0 0;0 -0.601815 -0.798636]  CS0Pos=[]  CS0Rot=[]  CS1Pos=[0.278697 0 0.369834]  CS1Rot=[0 0.798636 -0.601815;1 0 0;0 -0.601815 -0.798636]  CS2Pos=[0.28303 0.0011 0.375585]  CS2Rot=[1 0 0;0 1 0;0 0 1]  CS3Pos=[0.0379706 0 0.0503802]  CS3Rot=[1 0 0;0 1 0;0 0 1]  CS4Pos=[]  CS4Rot=[]  CS5Pos=[]  CS5Rot=[]  CS6Pos=[]  CS6Rot=[]  CS7Pos=[]  CS7Rot=[]  CS8Pos=[]  CS8Rot=[]  CS9Pos=[]  CS9Rot=[]  CS10Pos=[]  CS10Rot=[]  CS11Pos=[]  CS11Rot=[]  CS12Pos=[]  CS12Rot=[]  CS13Pos=[]  CS13Rot=[]  CS14Pos=[]  CS14Rot=[]  CS15Pos=[]  CS15Rot=[]  CS16Pos=[]  CS16Rot=[]  CS17Pos=[]  CS17Rot=[]  CS18Pos=[]  CS18Rot=[]  CS19Pos=[]  CS19Rot=[]  CS20Pos=[]  CS20Rot=[]
  tag scope: theta1_l=global, theta1_r=global, theta2_l=global, theta2_r=global, theta3_l=global, theta3_r=global
  wires:
  [tau1_r] -> Joint Actuator1/1
  Joint Sensor3/1 -> [theta2_r]
  Joint Sensor1/1 -> [theta3_r]
  [theta1_r] -> To Workspace1/1, Scope12/1
  [theta2_r] -> To Workspace2/1, Scope1/1
  [tau2_r] -> Joint Actuator2/1
  Joint Sensor2/1 -> [theta1_r]
  [theta3_r] -> To Workspace3/1, Scope2/1
  [tau3_r] -> Joint Actuator3/1
  [theta1_l] -> To Workspace8/1, Scope8/1
  [theta2_l] -> To Workspace9/1, Scope7/1
  [theta3_l] -> To Workspace10/1, Scope9/1
  Joint Sensor9/1 -> [theta1_l]
  [tau1_l_link] -> Joint Actuator8/1
  Joint Sensor10/1 -> [theta2_l]
  [tau2_l_link] -> Joint Actuator9/1
  [tau3_l_link] -> Joint Actuator4/1
  Joint Sensor4/1 -> [theta3_l]
  connections:
  link1_l/RConn1 -- Revolute7/LConn1
  base_right/LConn2 -- Revolute4/LConn1
  base_left/RConn1 -- Revolute8/LConn1
  Revolute5/LConn1 -- link1_r/RConn1
  Revolute8/RConn1 -- link1_l/LConn1
  Weld/LConn1 -- tool_adaptor_r/RConn1
  Weld/RConn1 -- tool_shaft_r/LConn1
  link2_r/LConn1 -- Revolute5/RConn1
  Prismatic1/RConn1 -- tool_adaptor_r/LConn1
  link2_r/RConn1 -- Prismatic1/LConn1
  base_right/LConn1 -- base_left/LConn1
  Revolute4/LConn2 -- Joint Sensor2/LConn1
  Prismatic1/LConn2 -- Joint Sensor1/LConn1
  Revolute4/RConn1 -- link1_r/LConn1
  Revolute5/RConn2 -- Joint Actuator2/RConn1
  Prismatic1/RConn2 -- Joint Actuator3/RConn1
  Revolute5/LConn3 -- Joint Initial Condition2/RConn1
  Revolute4/LConn3 -- Joint Initial Condition1/RConn1
  Revolute5/LConn2 -- Joint Sensor3/LConn1
  Revolute4/RConn2 -- Joint Actuator1/RConn1
  Prismatic1/LConn3 -- Joint Initial Condition3/RConn1
  Revolute8/LConn3 -- Joint Initial Condition8/RConn1
  Revolute8/RConn2 -- Joint Actuator8/RConn1
  Revolute7/RConn2 -- Joint Actuator9/RConn1
  Revolute7/LConn2 -- Joint Sensor10/LConn1
  Revolute7/LConn3 -- Joint Initial Condition9/RConn1
  Revolute8/LConn2 -- Joint Sensor9/LConn1
  Prismatic2/RConn2 -- Joint Actuator4/RConn1
  Prismatic2/RConn1 -- tool_adaptor_l/RConn1
  Prismatic2/LConn2 -- Joint Sensor4/LConn1
  Prismatic2/LConn3 -- Joint Initial Condition4/RConn1
  Revolute7/RConn1 -- link2_l1/LConn1
  link2_l1/RConn1 -- Prismatic2/LConn1

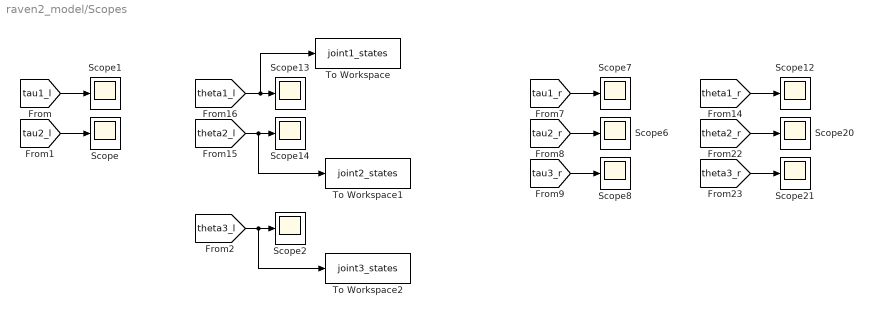
== system raven2_model/Scopes ==
  Scope{,1..2,6..8,12..14,20..21} (11 alike) : Scope
  To Workspace : ToWorkspace  VariableName=joint1_states  SaveFormat=Timeseries  SampleTime=-1
  To Workspace1 : ToWorkspace  VariableName=joint2_states  SaveFormat=Timeseries  SampleTime=-1
  To Workspace2 : ToWorkspace  VariableName=joint3_states  SaveFormat=Timeseries  SampleTime=-1
  wires:
  [tau2_l] -> Scope/1
  [tau1_l] -> Scope1/1
  [tau2_r] -> Scope6/1
  [tau1_r] -> Scope7/1
  [tau3_r] -> Scope8/1
  [theta1_r] -> Scope12/1
  [theta1_l] -> To Workspace/1, Scope13/1
  [theta2_l] -> To Workspace1/1, Scope14/1
  [theta2_r] -> Scope20/1
  [theta3_r] -> Scope21/1
  [theta3_l] -> To Workspace2/1, Scope2/1

== system raven2_model/Joint_Control/left_arm_control_command_signal ==

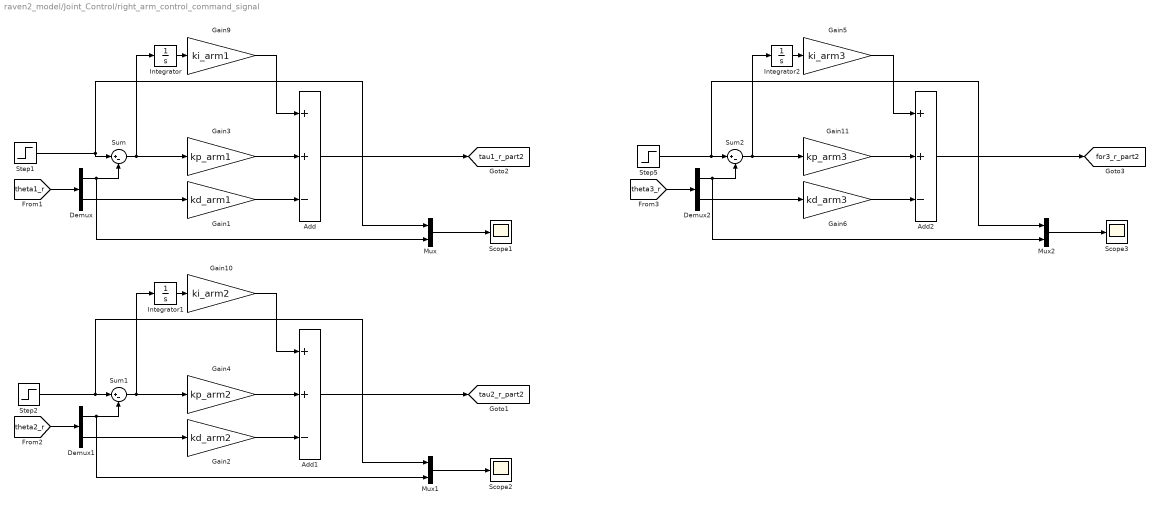
== system raven2_model/Joint_Control/right_arm_control_command_signal ==
  Add : Sum  Inputs=++-
  Add1 : Sum  Inputs=++-
  Add2 : Sum  Inputs=++-
  Demux : Demux  Outputs=2
  Demux1 : Demux  Outputs=2
  Demux2 : Demux  Outputs=2
  Gain1 : Gain  Gain=kd_arm1
  Gain10 : Gain  Gain=ki_arm2
  Gain11 : Gain  Gain=kp_arm3
  Gain2 : Gain  Gain=kd_arm2
  Gain3 : Gain  Gain=kp_arm1
  Gain4 : Gain  Gain=kp_arm2
  Gain5 : Gain  Gain=ki_arm3
  Gain6 : Gain  Gain=kd_arm3
  Gain9 : Gain  Gain=ki_arm1
  Integrator : Integrator
  Integrator1 : Integrator
  Integrator2 : Integrator
  Mux : Mux  Inputs=2
  Mux1 : Mux  Inputs=2
  Mux2 : Mux  Inputs=2
  Scope1 : Scope
  Scope2 : Scope
  Scope3 : Scope
  Step1 : Step  Time=0  Before=theta1_0_r  After=theta1_d_r  SampleTime=0
  Step2 : Step  Time=0  Before=theta2_0_r  After=theta2_d_r  SampleTime=0
  Step5 : Step  Time=0  Before=theta3_0_r  After=theta3_d_r  SampleTime=0
  Sum : Sum  Inputs=|+-
  Sum1 : Sum  Inputs=|+-
  Sum2 : Sum  Inputs=|+-
  tag scope: for3_r_part2=global, tau1_r_part2=global, tau2_r_part2=global
  wires:
  [theta1_r] -> Demux/1
  Demux/2 -> Gain1/1
  Add/1 -> [tau1_r_part2]
  Step1/1 -> Sum/1, Mux/1
  Demux/1 -> Mux/2, Sum/2
  Mux/1 -> Scope1/1
  Sum/1 -> Gain3/1, Integrator/1
  Integrator/1 -> Gain9/1
  Gain1/1 -> Add/3
  Gain3/1 -> Add/2
  Gain9/1 -> Add/1
  [theta2_r] -> Demux1/1
  Demux1/2 -> Gain2/1
  Add1/1 -> [tau2_r_part2]
  Step2/1 -> Mux1/1, Sum1/1
  Demux1/1 -> Mux1/2, Sum1/2
  Mux1/1 -> Scope2/1
  Sum1/1 -> Gain4/1, Integrator1/1
  Integrator1/1 -> Gain10/1
  Gain2/1 -> Add1/3
  Gain4/1 -> Add1/2
  Gain10/1 -> Add1/1
  [theta3_r] -> Demux2/1
  Demux2/2 -> Gain6/1
  Add2/1 -> [for3_r_part2]
  Step5/1 -> Mux2/1, Sum2/1
  Demux2/1 -> Mux2/2, Sum2/2
  Mux2/1 -> Scope3/1
  Sum2/1 -> Gain11/1, Integrator2/1
  Integrator2/1 -> Gain5/1
  Gain6/1 -> Add2/3
  Gain11/1 -> Add2/2
  Gain5/1 -> Add2/1

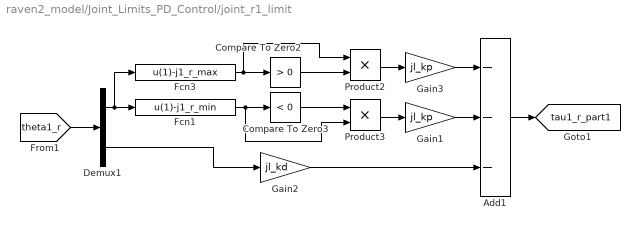
== system raven2_model/Joint_Limits_PD_Control/joint_r1_limit ==
  Add1 : Sum  Inputs=---
  Compare To Zero2 : simulink/Logic and Bit Operations/Compare To Zero  relop=>  OutDataTypeStr=boolean
  Compare To Zero3 : simulink/Logic and Bit Operations/Compare To Zero  relop=<  OutDataTypeStr=boolean
  Demux1 : Demux  Outputs=2
  Fcn1 : Fcn  Expr=u(1)-j1_r_min
  Fcn3 : Fcn  Expr=u(1)-j1_r_max
  Gain1 : Gain  Gain=jl_kp
  Gain2 : Gain  Gain=jl_kd
  Gain3 : Gain  Gain=jl_kp
  Product2 : Product
  Product3 : Product
  tag scope: tau1_r_part1=global
  wires:
  Gain3/1 -> Add1/1
  Fcn3/1 -> Product2/1, Compare To Zero2/1
  Gain1/1 -> Add1/2
  Add1/1 -> [tau1_r_part1]
  Product2/1 -> Gain3/1
  Product3/1 -> Gain1/1
  Compare To Zero3/1 -> Product3/1
  Demux1/2 -> Gain2/1
  Fcn1/1 -> Product3/2, Compare To Zero3/1
  [theta1_r] -> Demux1/1
  Gain2/1 -> Add1/3
  Compare To Zero2/1 -> Product2/2
  Demux1/1 -> Fcn1/1, Fcn3/1

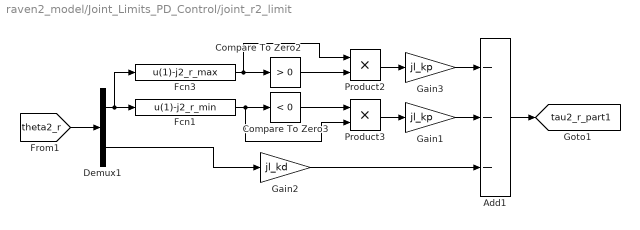
== system raven2_model/Joint_Limits_PD_Control/joint_r2_limit ==
  Add1 : Sum  Inputs=---
  Compare To Zero2 : simulink/Logic and Bit Operations/Compare To Zero  relop=>  OutDataTypeStr=boolean
  Compare To Zero3 : simulink/Logic and Bit Operations/Compare To Zero  relop=<  OutDataTypeStr=boolean
  Demux1 : Demux  Outputs=2
  Fcn1 : Fcn  Expr=u(1)-j2_r_min
  Fcn3 : Fcn  Expr=u(1)-j2_r_max
  Gain1 : Gain  Gain=jl_kp
  Gain2 : Gain  Gain=jl_kd
  Gain3 : Gain  Gain=jl_kp
  Product2 : Product
  Product3 : Product
  tag scope: tau2_r_part1=global
  wires:
  Gain3/1 -> Add1/1
  Fcn3/1 -> Product2/1, Compare To Zero2/1
  Gain1/1 -> Add1/2
  Add1/1 -> [tau2_r_part1]
  Product2/1 -> Gain3/1
  Product3/1 -> Gain1/1
  Compare To Zero3/1 -> Product3/1
  Demux1/2 -> Gain2/1
  Fcn1/1 -> Product3/2, Compare To Zero3/1
  [theta2_r] -> Demux1/1
  Gain2/1 -> Add1/3
  Compare To Zero2/1 -> Product2/2
  Demux1/1 -> Fcn1/1, Fcn3/1

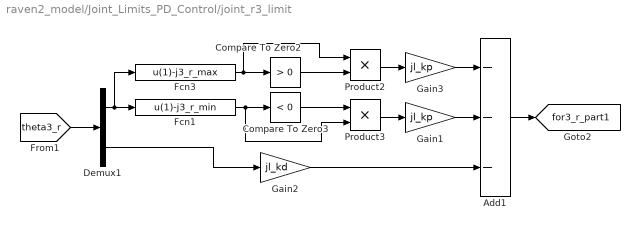
== system raven2_model/Joint_Limits_PD_Control/joint_r3_limit ==
  Add1 : Sum  Inputs=---
  Compare To Zero2 : simulink/Logic and Bit Operations/Compare To Zero  relop=>  OutDataTypeStr=boolean
  Compare To Zero3 : simulink/Logic and Bit Operations/Compare To Zero  relop=<  OutDataTypeStr=boolean
  Demux1 : Demux  Outputs=2
  Fcn1 : Fcn  Expr=u(1)-j3_r_min
  Fcn3 : Fcn  Expr=u(1)-j3_r_max
  Gain1 : Gain  Gain=jl_kp
  Gain2 : Gain  Gain=jl_kd
  Gain3 : Gain  Gain=jl_kp
  Product2 : Product
  Product3 : Product
  tag scope: for3_r_part1=global
  wires:
  Gain3/1 -> Add1/1
  Fcn3/1 -> Product2/1, Compare To Zero2/1
  Gain1/1 -> Add1/2
  Add1/1 -> [for3_r_part1]
  Product2/1 -> Gain3/1
  Product3/1 -> Gain1/1
  Compare To Zero3/1 -> Product3/1
  Demux1/2 -> Gain2/1
  Fcn1/1 -> Product3/2, Compare To Zero3/1
  [theta3_r] -> Demux1/1
  Gain2/1 -> Add1/3
  Compare To Zero2/1 -> Product2/2
  Demux1/1 -> Fcn1/1, Fcn3/1

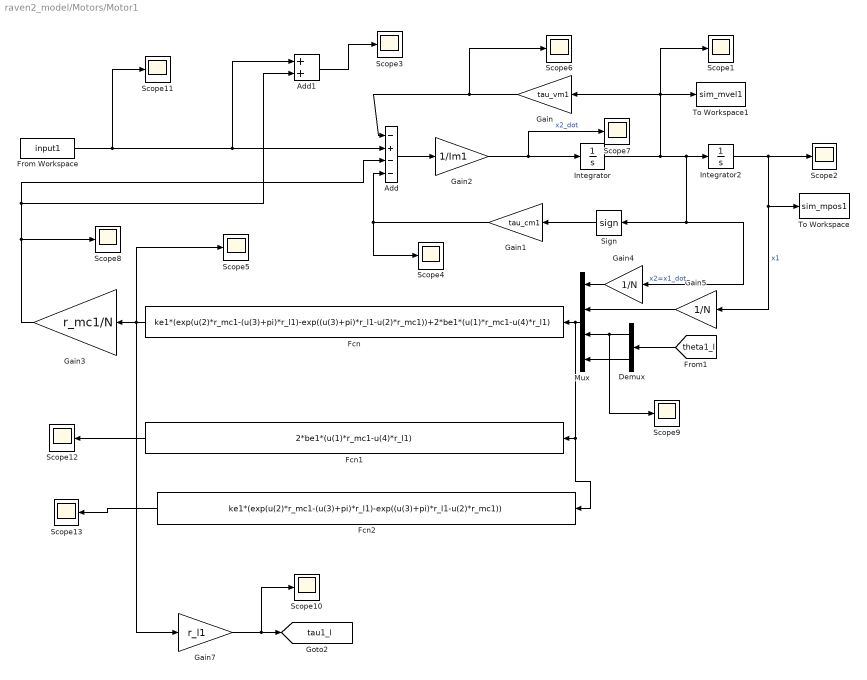
== system raven2_model/Motors/Motor1 ==
  Add : Sum  Inputs=-+--
  Add1 : Sum
  Demux : Demux  Outputs=2
  Fcn : Fcn  Expr=ke1*(exp(u(2)*r_mc1-(u(3)+pi)*r_l1)-exp((u(3)+pi)*r_l1-u(2)*r_mc1))+2*be1*(u(1)*r_mc1-u(4)*r_l1)
  Fcn1 : Fcn  Expr=2*be1*(u(1)*r_mc1-u(4)*r_l1)
  Fcn2 : Fcn  Expr=ke1*(exp(u(2)*r_mc1-(u(3)+pi)*r_l1)-exp((u(3)+pi)*r_l1-u(2)*r_mc1))
  From Workspace : FromWorkspace  VariableName=input1  SampleTime=0
  Gain : Gain  Gain=tau_vm1
  Gain1 : Gain  Gain=tau_cm1
  Gain2 : Gain  Gain=1/Im1
  Gain3 : Gain  Gain=r_mc1/N
  Gain4 : Gain  Gain=1/N
  Gain5 : Gain  Gain=1/N
  Gain7 : Gain  Gain=r_l1
  Integrator : Integrator  InitialCondition=m1_vel_ini
  Integrator2 : Integrator  InitialCondition=m1_pos_ini
  Mux : Mux
  Scope{1..13} (13 alike) : Scope
  Sign : Signum  ZeroCross=off
  To Workspace : ToWorkspace  VariableName=sim_mpos1  SaveFormat=Timeseries  SampleTime=-1
  To Workspace1 : ToWorkspace  VariableName=sim_mvel1  SaveFormat=Timeseries  SampleTime=-1
  tag scope: tau1_l=global
  wires:
  Integrator/1 -> Scope1/1, To Workspace1/1, Gain/1, Gain4/1, Sign/1, Integrator2/1  "x2=x1_dot"
  Integrator2/1 -> To Workspace/1, Gain5/1, Scope2/1  "x1"
  Sign/1 -> Gain1/1
  Gain5/1 -> Mux/2
  Mux/1 -> Fcn2/1, Fcn1/1, Fcn/1
  Gain1/1 -> Add/4, Scope4/1
  Gain3/1 -> Scope8/1, Add1/2, Add/3
  Gain7/1 -> [tau1_l], Scope10/1
  Fcn/1 -> Gain7/1, Scope5/1, Gain3/1
  Demux/2 -> Mux/4
  Gain4/1 -> Mux/1
  Gain/1 -> Scope6/1, Add/1
  [theta1_l] -> Demux/1
  Gain2/1 -> Scope7/1, Integrator/1  "x2_dot"
  Demux/1 -> Scope9/1, Mux/3
  Add/1 -> Gain2/1
  From Workspace/1 -> Scope11/1, Add1/1, Add/2
  Fcn1/1 -> Scope12/1
  Fcn2/1 -> Scope13/1
  Add1/1 -> Scope3/1

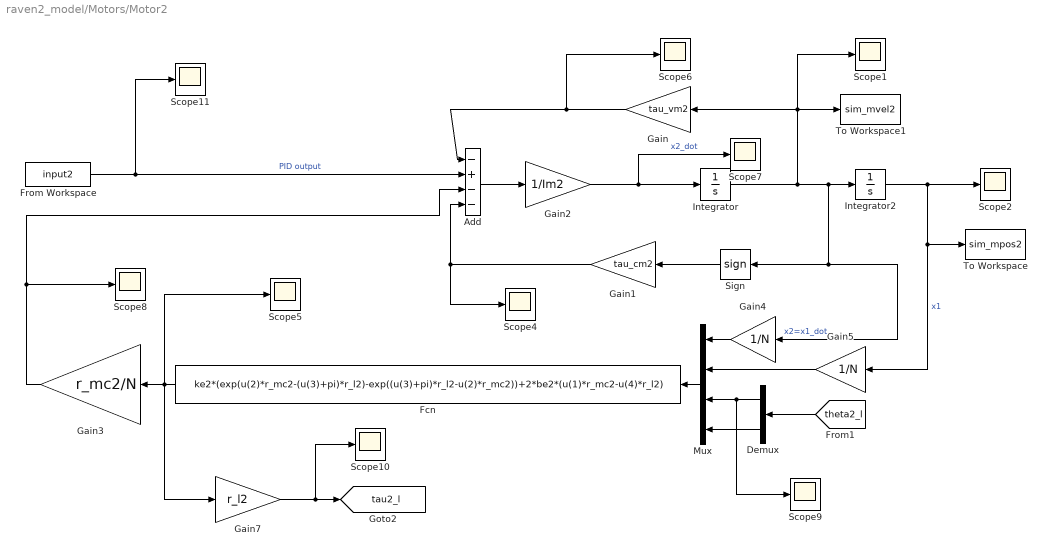
== system raven2_model/Motors/Motor2 ==
  Add : Sum  Inputs=-+--
  Demux : Demux  Outputs=2
  Fcn : Fcn  Expr=ke2*(exp(u(2)*r_mc2-(u(3)+pi)*r_l2)-exp((u(3)+pi)*r_l2-u(2)*r_mc2))+2*be2*(u(1)*r_mc2-u(4)*r_l2)
  From Workspace : FromWorkspace  VariableName=input2  SampleTime=0
  Gain : Gain  Gain=tau_vm2
  Gain1 : Gain  Gain=tau_cm2
  Gain2 : Gain  Gain=1/Im2
  Gain3 : Gain  Gain=r_mc2/N
  Gain4 : Gain  Gain=1/N
  Gain5 : Gain  Gain=1/N
  Gain7 : Gain  Gain=r_l2
  Integrator : Integrator  InitialCondition=m2_vel_ini
  Integrator2 : Integrator  InitialCondition=m2_pos_ini
  Mux : Mux
  Scope{1..2,4..11} (10 alike) : Scope
  Sign : Signum  ZeroCross=off
  To Workspace : ToWorkspace  VariableName=sim_mpos2  SaveFormat=Timeseries  SampleTime=-1
  To Workspace1 : ToWorkspace  VariableName=sim_mvel2  SaveFormat=Timeseries  SampleTime=-1
  tag scope: tau2_l=global
  wires:
  Integrator/1 -> Scope1/1, To Workspace1/1, Gain/1, Gain4/1, Sign/1, Integrator2/1  "x2=x1_dot"
  Integrator2/1 -> To Workspace/1, Gain5/1, Scope2/1  "x1"
  Sign/1 -> Gain1/1
  Gain5/1 -> Mux/2
  Mux/1 -> Fcn/1
  Gain1/1 -> Add/4, Scope4/1
  Gain3/1 -> Scope8/1, Add/3
  Gain7/1 -> [tau2_l], Scope10/1
  Fcn/1 -> Gain7/1, Scope5/1, Gain3/1
  Demux/2 -> Mux/4
  Gain4/1 -> Mux/1
  Gain/1 -> Scope6/1, Add/1
  [theta2_l] -> Demux/1
  Gain2/1 -> Scope7/1, Integrator/1  "x2_dot"
  Demux/1 -> Scope9/1, Mux/3
  Add/1 -> Gain2/1
  From Workspace/1 -> Add/2, Scope11/1  "PID output"

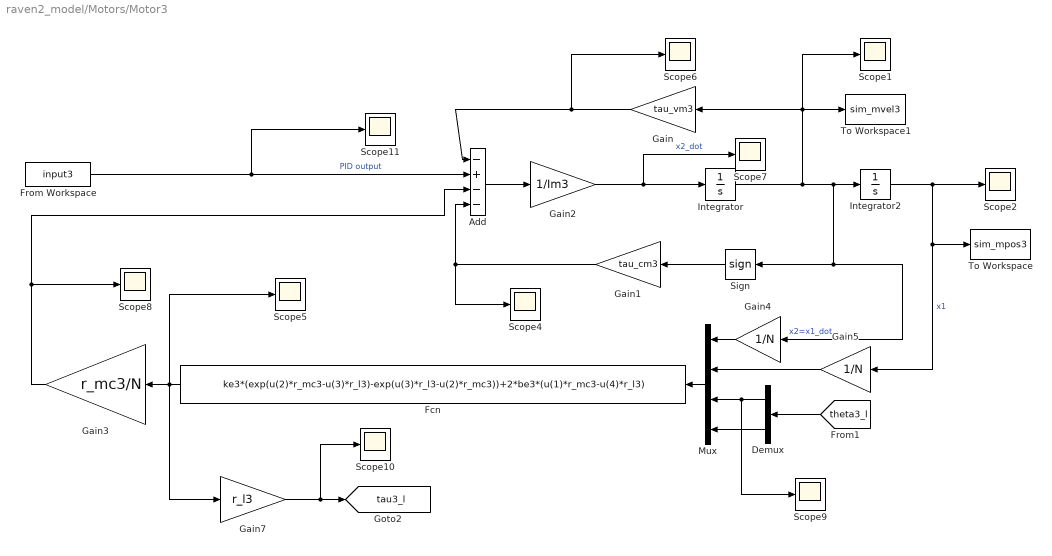
== system raven2_model/Motors/Motor3 ==
  Add : Sum  Inputs=-+--
  Demux : Demux  Outputs=2
  Fcn : Fcn  Expr=ke3*(exp(u(2)*r_mc3-u(3)*r_l3)-exp(u(3)*r_l3-u(2)*r_mc3))+2*be3*(u(1)*r_mc3-u(4)*r_l3)
  From Workspace : FromWorkspace  VariableName=input3  SampleTime=0
  Gain : Gain  Gain=tau_vm3
  Gain1 : Gain  Gain=tau_cm3
  Gain2 : Gain  Gain=1/Im3
  Gain3 : Gain  Gain=r_mc3/N
  Gain4 : Gain  Gain=1/N
  Gain5 : Gain  Gain=1/N
  Gain7 : Gain  Gain=r_l3
  Integrator : Integrator  InitialCondition=m3_vel_ini
  Integrator2 : Integrator  InitialCondition=m3_pos_ini
  Mux : Mux
  Scope{1..2,4..11} (10 alike) : Scope
  Sign : Signum  ZeroCross=off
  To Workspace : ToWorkspace  VariableName=sim_mpos3  SaveFormat=Timeseries  SampleTime=-1
  To Workspace1 : ToWorkspace  VariableName=sim_mvel3  SaveFormat=Timeseries  SampleTime=-1
  tag scope: tau3_l=global
  wires:
  Integrator/1 -> Scope1/1, To Workspace1/1, Gain/1, Gain4/1, Sign/1, Integrator2/1  "x2=x1_dot"
  Integrator2/1 -> To Workspace/1, Gain5/1, Scope2/1  "x1"
  Sign/1 -> Gain1/1
  Gain5/1 -> Mux/2
  Mux/1 -> Fcn/1
  Gain1/1 -> Add/4, Scope4/1
  Gain3/1 -> Scope8/1, Add/3
  Gain7/1 -> [tau3_l], Scope10/1
  Fcn/1 -> Gain7/1, Scope5/1, Gain3/1
  Demux/2 -> Mux/4
  Gain4/1 -> Mux/1
  Gain/1 -> Scope6/1, Add/1
  [theta3_l] -> Demux/1
  Gain2/1 -> Scope7/1, Integrator/1  "x2_dot"
  Demux/1 -> Scope9/1, Mux/3
  Add/1 -> Gain2/1
  From Workspace/1 -> Add/2, Scope11/1  "PID output"

== system raven2_model/Robot_Mechanics/base_left ==
  Weld1 : mblibv1/Joints/Weld  LConnTagsString=__newl0  RConnTagsString=__newr0  UpdateFromCAD=on  NumSAPorts=0  CutJoint=off  MarkAsCut=off  Primitives=weld  PrimitiveProps=W$WORLD$[0.57735,0.57735,0.57735]$weld  DialogClass=JointBlock  WAxis=[0.57735,0.57735,0.57735]
  base_l-1 : mblibv1/Bodies/Body  LConnTagsString=CS2  RConnTagsString=CS3  UpdateFromCAD=on  DialogClass=MechanicalBodyBlock  Mass=0.00259737  MassUnits=kg  InertiaUnits=kg*m^2  Inertia=[1.48601e-05,4.37984e-06,1.41572e-06;4.37984e-06,2.15177e-05,-1.98455e-06;1.41572e-06,-1.98455e-06,3.16346e-05]  Shape=Cylinder  ShapeDims=[1 1]  ShapeUnits=m  ShapeUse=false  Density=1  DensityUnits=kg/m^3  DensityUse=false  GraphicsMode=GFXFILE  GraphicsFileName=full_robot - base_l-1.STL  BodyColorSelMode=COLORPALETTE  BodyColor=[0.247059;0.247059;0.247059]  AttachedToCS=CS1  CG=Right$CG$[-0.444677 0.0710164 0.00796487]$WORLD$WORLD$m$[1 0 0;0 1 0;0 0 1]$3x3 Transform$rad$WORLD$false$none  WorkingFrames=Right$CS1$[-0.506557 -0.150889 -0.323499]$WORLD$WORLD$m$[1 0 0;0 1 0;0 0 1]$3x3 Transform$rad$WORLD$false$none#Left$CS2$[0.1336 -0.0223119 -0.0261432]$WORLD$WORLD$m$[1 0 0;0 1 0;0 0 1]$3x3 Transform$rad$WORLD$true$none#Right$CS3$[-0.284078 0 0]$WORLD$WORLD$m$[1 0 0;0 1 0;0 0 1]$3x3 Transform$rad$WORLD$true$none  CGPos=[-0.444677 0.0710164 0.00796487]  CGRot=[1 0 0;0 1 0;0 0 1]  CS0Pos=[]  CS0Rot=[]  CS1Pos=[-0.506557 -0.150889 -0.323499]  CS1Rot=[1 0 0;0 1 0;0 0 1]  CS2Pos=[0.1336 -0.0223119 -0.0261432]  CS2Rot=[1 0 0;0 1 0;0 0 1]  CS3Pos=[-0.284078 0 0]  CS3Rot=[1 0 0;0 1 0;0 0 1]  CS4Pos=[]  CS4Rot=[]  CS5Pos=[]  CS5Rot=[]  CS6Pos=[]  CS6Rot=[]  CS7Pos=[]  CS7Rot=[]  CS8Pos=[]  CS8Rot=[]  CS9Pos=[]  CS9Rot=[]  CS10Pos=[]  CS10Rot=[]  CS11Pos=[]  CS11Rot=[]  CS12Pos=[]  CS12Rot=[]  CS13Pos=[]  CS13Rot=[]  CS14Pos=[]  CS14Rot=[]  CS15Pos=[]  CS15Rot=[]  CS16Pos=[]  CS16Rot=[]  CS17Pos=[]  CS17Rot=[]  CS18Pos=[]  CS18Rot=[]  CS19Pos=[]  CS19Rot=[]  CS20Pos=[]  CS20Rot=[]
  Conn1 : PMIOPort  Port=1  Side=Right
  Conn2 : PMIOPort  Port=2  Side=Left
  connections:
  Conn2/RConn1 -- Weld1/LConn1
  base_l-1/RConn1 -- Conn1/RConn1
  Weld1/RConn1 -- base_l-1/LConn1

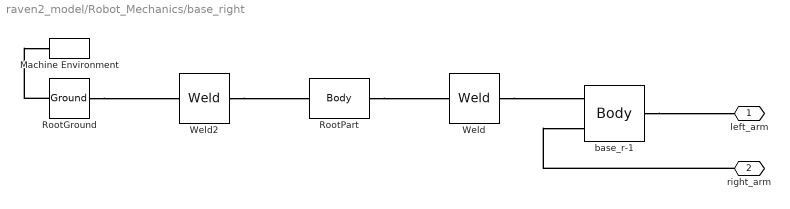
== system raven2_model/Robot_Mechanics/base_right ==
  Machine Environment : mblibv1/Bodies/Machine Environment  PortType=env  PhysicalDomain=Mechanical  DialogTemplateClass=MECH.MachineEnvironment  SyncWhenCopied=off  Gravity=gravity  GravityUnits=m/s^2  GravityAsSignal=off  Dimensionality=Auto-detect  AnalysisType=Forward dynamics  LinearAssemblyTolerance=1e-3  LinearAssemblyToleranceUnits=m  AngularAssemblyTolerance=1e-3  AngularAssemblyToleranceUnits=rad  ConstraintSolverType=Stabilizing  ConstraintRelTolerance=1e-4  ConstraintAbsTolerance=1e-4  UseRobustSingularityHandling=off  RedundancyAnalysisToleranceType=Automatically select tolerance  RedundancyAnalysisTolerance=1e-14  StatePerturbationType=Fixed  PerturbationSize=1e-5  VisualizeMachine=on  BodyVisualizationType=Use model default body geometries  BodyColorSelMode=Use model default  DefaultBodyColor=[1 0 0]
  RootGround : mblibv1/Bodies/Ground  UpdateFromCAD=on  LeftPortType=env  RightPortType=workingframe  PhysicalDomain=Mechanical  DialogClass=GroundBlock  CoordPosition=[-0.0533012,0.0536923,0.00289896]  CoordPositionUnits=m  StateVectorMgrId=1  MachineId=[2 0]  ShowEnvPort=on  ParameterChecksum=[3229275921, 2660409537, 479412719, 1714508742]  TopologyChecksum=[2751328460, 2190135854, 729012382, 2518639465]
  RootPart : mblibv1/Bodies/Body  LConnTagsString=CS3  RConnTagsString=CS2  UpdateFromCAD=on  DialogClass=MechanicalBodyBlock  Mass=0  MassUnits=kg  InertiaUnits=kg*m^2  Inertia=[0,0,0;0,0,0;0,0,0]  Shape=Cylinder  ShapeDims=[1 1]  ShapeUnits=m  ShapeUse=false  Density=1  DensityUnits=kg/m^3  DensityUse=false  GraphicsMode=MACHINE_DEFAULT  BodyColorSelMode=MACHINE_DEFAULT  BodyColor=[1;0;0]  AttachedToCS=CS1  CG=Right$CG$[-0.0533012 0.0536923 0.00289896]$WORLD$WORLD$m$[1 0 0;0 1 0;0 0 1]$3x3 Transform$rad$WORLD$false$none  WorkingFrames=Right$CS1$[0 0 0]$WORLD$WORLD$m$[1 0 0;0 1 0;0 0 1]$3x3 Transform$rad$WORLD$false$none#Right$CS2$[0.361877 0.0710923 0.00804081]$WORLD$WORLD$m$[1 0 0;0 1 0;0 0 1]$3x3 Transform$rad$WORLD$true$none#Left$CS3$[-0.0533012 0.0536923 0.00289896]$WORLD$WORLD$m$[1 0 0;0 1 0;0 0 1]$3x3 Transform$rad$WORLD$true$none  CGPos=[-0.0533012 0.0536923 0.00289896]  CGRot=[1 0 0;0 1 0;0 0 1]  CS0Pos=[]  CS0Rot=[]  CS1Pos=[0 0 0]  CS1Rot=[1 0 0;0 1 0;0 0 1]  CS2Pos=[0.361877 0.0710923 0.00804081]  CS2Rot=[1 0 0;0 1 0;0 0 1]  CS3Pos=[-0.0533012 0.0536923 0.00289896]  CS3Rot=[1 0 0;0 1 0;0 0 1]  CS4Pos=[]  CS4Rot=[]  CS5Pos=[]  CS5Rot=[]  CS6Pos=[]  CS6Rot=[]  CS7Pos=[]  CS7Rot=[]  CS8Pos=[]  CS8Rot=[]  CS9Pos=[]  CS9Rot=[]  CS10Pos=[]  CS10Rot=[]  CS11Pos=[]  CS11Rot=[]  CS12Pos=[]  CS12Rot=[]  CS13Pos=[]  CS13Rot=[]  CS14Pos=[]  CS14Rot=[]  CS15Pos=[]  CS15Rot=[]  CS16Pos=[]  CS16Rot=[]  CS17Pos=[]  CS17Rot=[]  CS18Pos=[]  CS18Rot=[]  CS19Pos=[]  CS19Rot=[]  CS20Pos=[]  CS20Rot=[]
  Weld : mblibv1/Joints/Weld  LConnTagsString=__newl0  RConnTagsString=__newr0  UpdateFromCAD=on  NumSAPorts=0  CutJoint=off  MarkAsCut=off  Primitives=weld  PrimitiveProps=W$WORLD$[0.57735,0.57735,0.57735]$weld  DialogClass=JointBlock  WAxis=[0.57735,0.57735,0.57735]
  Weld2 : mblibv1/Joints/Weld  LConnTagsString=__newl0  RConnTagsString=__newr0  UpdateFromCAD=on  NumSAPorts=0  CutJoint=off  MarkAsCut=off  Primitives=weld  PrimitiveProps=W$WORLD$[0.57735,0.57735,0.57735]$weld  DialogClass=JointBlock  WAxis=[0.57735,0.57735,0.57735]
  base_r-1 : mblibv1/Bodies/Body  LConnTagsString=CS2|CS3  RConnTagsString=CS4  UpdateFromCAD=on  DialogClass=MechanicalBodyBlock  Mass=0.00259661  MassUnits=kg  InertiaUnits=kg*m^2  Inertia=[1.48387e-05,1.43278e-06,4.39863e-06;1.43278e-06,3.16307e-05,-1.97705e-06;4.39863e-06,-1.97705e-06,2.14992e-05]  Shape=Cylinder  ShapeDims=[1 1]  ShapeUnits=m  ShapeUse=false  Density=1  DensityUnits=kg/m^3  DensityUse=false  GraphicsMode=GFXFILE  GraphicsFileName=full_robot - base_r-1.STL  BodyColorSelMode=COLORPALETTE  BodyColor=[0.247059;0.247059;0.247059]  AttachedToCS=CS1  CG=Right$CG$[0.361877 0.0710923 0.00804081]$WORLD$WORLD$m$[-1 0 0;0 0 1;0 1 0]$3x3 Transform$rad$WORLD$false$none  WorkingFrames=Right$CS1$[1.02617 0.370742 0.0607085]$WORLD$WORLD$m$[-1 0 0;0 0 1;0 1 0]$3x3 Transform$rad$WORLD$false$none#Left$CS2$[0.361877 0.0710923 0.00804081]$WORLD$WORLD$m$[1 0 0;0 1 0;0 0 1]$3x3 Transform$rad$WORLD$true$none#Left$CS3$[0.200746 0 0]$WORLD$WORLD$m$[1 0 0;0 1 0;0 0 1]$3x3 Transform$rad$WORLD$true$none#Right$CS4$[0.1336 -0.0223119 -0.0261432]$WORLD$WORLD$m$[1 0 0;0 1 0;0 0 1]$3x3 Transform$rad$WORLD$true$none  CGPos=[0.361877 0.0710923 0.00804081]  CGRot=[-1 0 0;0 0 1;0 1 0]  CS0Pos=[]  CS0Rot=[]  CS1Pos=[1.02617 0.370742 0.0607085]  CS1Rot=[-1 0 0;0 0 1;0 1 0]  CS2Pos=[0.361877 0.0710923 0.00804081]  CS2Rot=[1 0 0;0 1 0;0 0 1]  CS3Pos=[0.200746 0 0]  CS3Rot=[1 0 0;0 1 0;0 0 1]  CS4Pos=[0.1336 -0.0223119 -0.0261432]  CS4Rot=[1 0 0;0 1 0;0 0 1]  CS5Pos=[]  CS5Rot=[]  CS6Pos=[]  CS6Rot=[]  CS7Pos=[]  CS7Rot=[]  CS8Pos=[]  CS8Rot=[]  CS9Pos=[]  CS9Rot=[]  CS10Pos=[]  CS10Rot=[]  CS11Pos=[]  CS11Rot=[]  CS12Pos=[]  CS12Rot=[]  CS13Pos=[]  CS13Rot=[]  CS14Pos=[]  CS14Rot=[]  CS15Pos=[]  CS15Rot=[]  CS16Pos=[]  CS16Rot=[]  CS17Pos=[]  CS17Rot=[]  CS18Pos=[]  CS18Rot=[]  CS19Pos=[]  CS19Rot=[]  CS20Pos=[]  CS20Rot=[]
  left_arm : PMIOPort  Port=1  Side=Left
  right_arm : PMIOPort  Port=2  Side=Left
  connections:
  RootPart/RConn1 -- Weld/LConn1
  Weld2/RConn1 -- RootPart/LConn1
  Weld/RConn1 -- base_r-1/LConn1
  base_r-1/RConn1 -- left_arm/RConn1
  RootGround/RConn1 -- Weld2/LConn1
  right_arm/RConn1 -- base_r-1/LConn2
  RootGround/LConn1 -- Machine Environment/RConn1
